simulink model "fft8"  (R2026a)
settings: Solver=FixedStepDiscrete  StopTime=150  FixedStep=1
libraries: hdlsllib x1, dsphdlxfrm2 x1
settings Model: Creator=KoayXianCong  LastModifiedBy=KoayXianCong

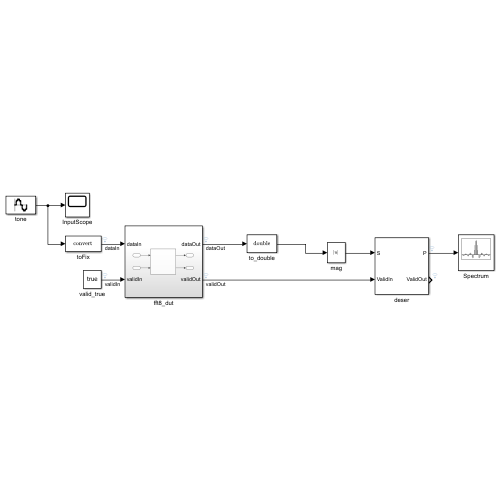
[thumbnail: Simulink's stored preview of the top-level diagram]
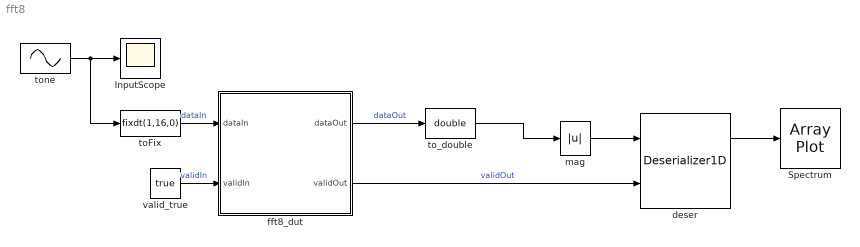
== system fft8 ==
  InputScope : Scope
      settings: ActiveDisplayYMinimum=-1  ActiveDisplayYMaximum=1
  Spectrum : ArrayPlot  WindowPosition=[368.000000,182.000000,800.000000,500.000000,]  ScopeFrameLocation=window  Title=FFT magnitude spectrum (bins 0-7)  YLabel=|FFT|  YLimits=[-500 4500]
  deser : hdlsllib/HDL Operations/Deserializer1D  Ratio=8  IdleCycles=0  InitialCondition=0  startIn=off  validIn=on  validOut=on  inputDataDimensions=-1  inputSampleTime=-1  inputSignalType=auto
  fft8_dut : Subsystem
  mag : Abs  SaturateOnIntegerOverflow=off
  toFix : DataTypeConversion  OutDataTypeStr=fixdt(1,16,0)  RndMeth=Nearest  SaturateOnIntegerOverflow=off
  to_double : DataTypeConversion  OutDataTypeStr=double  SaturateOnIntegerOverflow=off  RndMeth=Floor
  tone : Sin  Amplitude=1000  Frequency=1.5707963267948966  Phase=1.5707963267948966  SampleTime=1
  valid_true : Constant  Value=true  OutDataTypeStr=boolean  SampleTime=1
  wires:
  tone/1 -> toFix/1, InputScope/1
  valid_true/1 -> fft8_dut/2(validIn)  "validIn"
  toFix/1 -> fft8_dut/1(dataIn)  "dataIn"
  fft8_dut/2(validOut) -> deser/2  "validOut"
  fft8_dut/1(dataOut) -> to_double/1  "dataOut"
  to_double/1 -> mag/1
  mag/1 -> deser/1
  deser/1 -> Spectrum/1

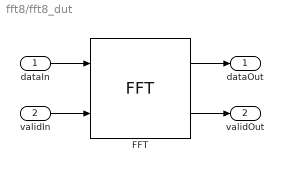
== system fft8/fft8_dut ==
  dataIn : Inport
  validIn : Inport  Port=2
  FFT : dsphdlxfrm2/FFT  Architecture=Streaming Radix 2^2  FFTLengthSource=Property  FFTLength=8  FFTLengthMax=1024  ComplexMultiplication=Use 4 multipliers and 2 adders  BitReversedOutput=off  BitReversedInput=off  Normalize=off  SimulateUsing=Code generation  RoundingMethod=Floor  ResetInputPort=off  StartOutputPort=off  EndOutputPort=off
  dataOut : Outport
  validOut : Outport  Port=2
  wires:
  dataIn/1 -> FFT/1
  FFT/2 -> validOut/1
  FFT/1 -> dataOut/1
  validIn/1 -> FFT/2
